simulink model "ABCDDiscreteModel_OptimalControlIntegral_Obs_mdl"  (Simulink 6.0)
settings: Solver=FixedStepDiscrete  StartTime=0.0  StopTime=10.0  FixedStep=Ts  RelTol=1e-3
values from neighbouring files (symbols this model uses):
  H = Ki(n+1)    [TSC150715ProvaMatlab.m]
  K = Ki(1:n)    [TSC150715ProvaMatlab.m]
  L = -acker(Az',Cz',[0 0 0])'    [TSC150715ProvaMatlab.m]
  Ts = 0.01    [TSC150715ProvaMatlab.m]
  X0 = [0;0;0]    [TSC150715ProvaMatlab.m]
  yp = 12    [TSC150715ProvaMatlab.m]
undefined symbols (not defined in the file or in its folder): Az, Bz, Cz, DiscIntNeverNeededParam
settings Model: Creator=lbiagiotti  LastModifiedBy=Biagio
settings OptimizationCC: InlineInvariantSignals=off  InitFltsAndDblsToZero=off
settings DebuggingCC: SignalResolutionControl=UseLocalSettings  FcnCallInpInsideContextMsg=Use local settings  StrictBusMsg=Warning
settings HardwareCC: TargetHWDeviceType=32-bit Generic

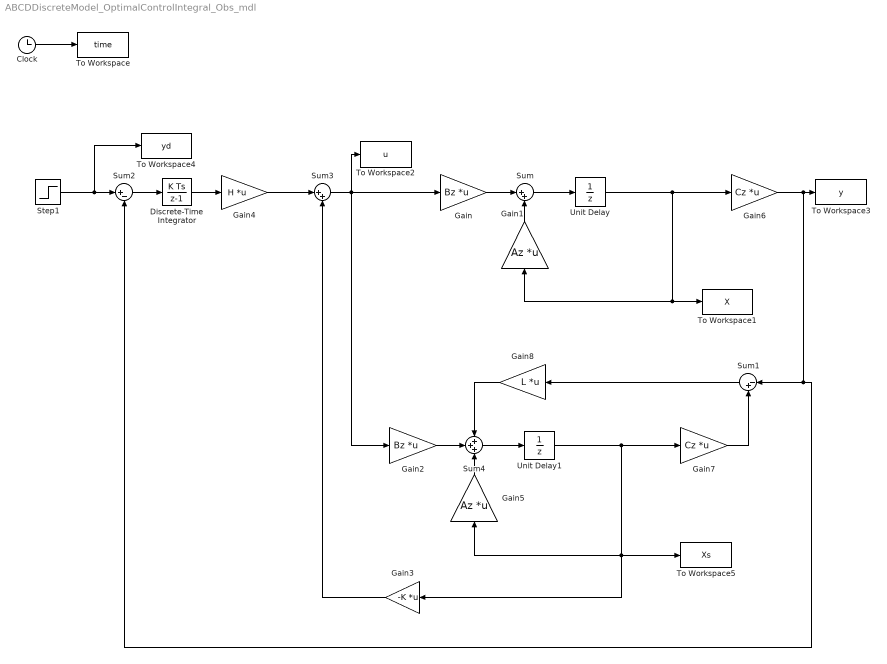
== system ABCDDiscreteModel_OptimalControlIntegral_Obs_mdl ==
  Clock : Clock
  Discrete-Time Integrator : DiscreteIntegrator  SampleTime=Ts  ICPrevOutput=DiscIntNeverNeededParam  ICPrevScaledInput=DiscIntNeverNeededParam
  Gain : Gain  Gain=Bz  Multiplication=Matrix(K*u)
  Gain1 : Gain  Orientation=up  Gain=Az  Multiplication=Matrix(K*u)
  Gain2 : Gain  Gain=Bz  Multiplication=Matrix(K*u)
  Gain3 : Gain  Orientation=left  Gain=-K  Multiplication=Matrix(K*u)
  Gain4 : Gain  Gain=H  Multiplication=Matrix(K*u)
  Gain5 : Gain  Orientation=up  Gain=Az  Multiplication=Matrix(K*u)
  Gain6 : Gain  Gain=Cz  Multiplication=Matrix(K*u)
  Gain7 : Gain  Gain=Cz  Multiplication=Matrix(K*u)
  Gain8 : Gain  Orientation=left  Gain=L  Multiplication=Matrix(K*u)
  Step1 : Step  After=yp  SampleTime=0
  Sum : Sum  Inputs=|++
  Sum1 : Sum  Orientation=left  Inputs=|-+
  Sum2 : Sum  Inputs=|+-
  Sum3 : Sum  Inputs=|++
  Sum4 : Sum  Inputs=+++
  To Workspace : ToWorkspace  VariableName=time  SampleTime=-1
  To Workspace1 : ToWorkspace  VariableName=X  SampleTime=-1
  To Workspace2 : ToWorkspace  VariableName=u  SampleTime=-1
  To Workspace3 : ToWorkspace  VariableName=y  SampleTime=-1
  To Workspace4 : ToWorkspace  VariableName=yd  SampleTime=-1
  To Workspace5 : ToWorkspace  VariableName=Xs  SampleTime=-1
  Unit Delay : UnitDelay  X0=X0  SampleTime=Ts
  Unit Delay1 : UnitDelay  SampleTime=Ts
  wires:
  Step1/1 -> To Workspace4/1, Sum2/1
  Clock/1 -> To Workspace/1
  Discrete-Time Integrator/1 -> Gain4/1
  Sum2/1 -> Discrete-Time Integrator/1
  Gain3/1 -> Sum3/2
  Sum3/1 -> Gain2/1, Gain/1, To Workspace2/1
  Sum/1 -> Unit Delay/1
  Unit Delay/1 -> Gain6/1, Gain1/1, To Workspace1/1
  Gain4/1 -> Sum3/1
  Gain6/1 -> To Workspace3/1, Sum2/2, Sum1/1
  Gain/1 -> Sum/1
  Gain1/1 -> Sum/2
  Sum4/1 -> Unit Delay1/1
  Unit Delay1/1 -> Gain7/1, Gain3/1, To Workspace5/1, Gain5/1
  Gain2/1 -> Sum4/2
  Gain5/1 -> Sum4/3
  Gain8/1 -> Sum4/1
  Sum1/1 -> Gain8/1
  Gain7/1 -> Sum1/2
